simulink model "Cinematica_JA_reducido"  (Simulink 7.7)
settings: Solver=ode45  StartTime=0.0  StopTime=inf  RelTol=1e-3
libraries: vrlib x1
settings Model: Creator=JohnConstantine  LastModifiedBy=JohnConstantine

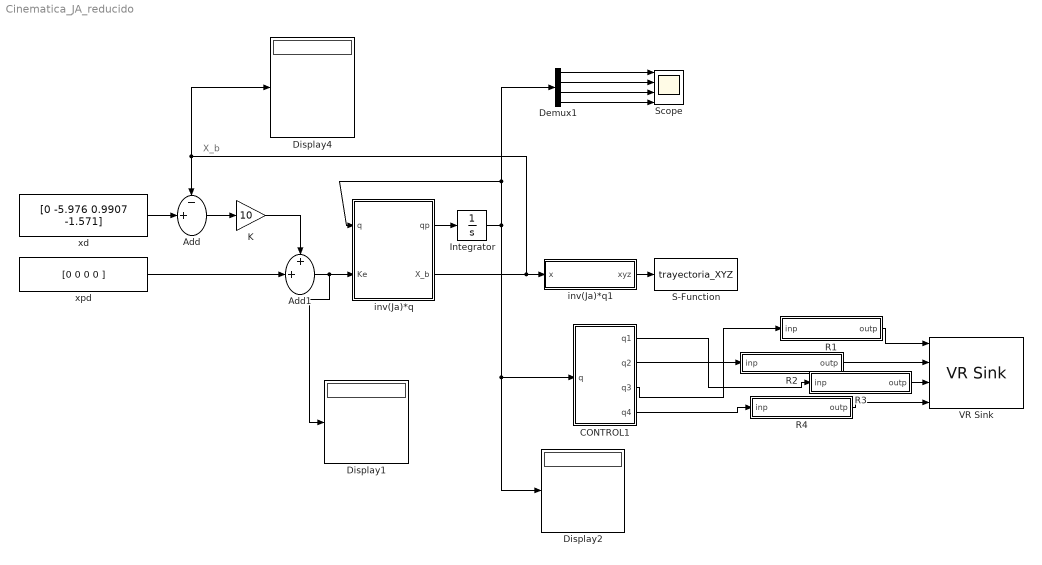
== system Cinematica_JA_reducido ==
  note: X_b
  Add : Sum  Inputs=-+|
  Add1 : Sum  Inputs=++|
  CONTROL1 : Stateflow chart  TreatAsAtomicUnit=on
  Demux1 : Demux
  Display1 : Display
  Display2 : Display
  Display4 : Display
  Integrator : Integrator  InitialCondition=[.001 .001 .001 .001]
  K : Gain  Gain=10
  R1 : Stateflow chart  TreatAsAtomicUnit=on
  R2 : Stateflow chart  TreatAsAtomicUnit=on
  R3 : Stateflow chart  TreatAsAtomicUnit=on
  R4 : Stateflow chart  TreatAsAtomicUnit=on
  S-Function : S-Function  FunctionName=trayectoria_XYZ  Parameters=[-7 7 -7 7 -7 7]  EnableBusSupport=off
  Scope : Scope  NumInputPorts=4
      settings: YMin=-0.2~0~0~-0.5  YMax=0.9~2.25~2~0.5
  VR Sink : vrlib/VR Sink  SampleTime=0.1  ViewEnable=on  RemoteChange=off  RemoteView=on  FieldsWritten=Q1.translation.3.1.1.double#Q2.rotation.4.1.1.double#Q3.rotation.4.1.1.double#Q4.rotation.4.1.1.double  WorldFileName=DedoCAD.WRL  AutoView=off  VideoDimensions=[]
  inv(Ja)*q : Stateflow chart  TreatAsAtomicUnit=on
  inv(Ja)*q1 : Stateflow chart  TreatAsAtomicUnit=on
  xd : Constant  Value=[0 -5.976 0.9907 -1.571]
  xpd : Constant  Value=[0 0 0 0 ]
  wires:
  Add/1 -> K/1
  xd/1 -> Add/2
  K/1 -> Add1/1
  xpd/1 -> Add1/2
  Add1/1 -> Display1/1, inv(Ja)*q/2(Ke)
  Integrator/1 -> inv(Ja)*q/1(q), Demux1/1, CONTROL1/1(q), Display2/1
  inv(Ja)*q/2(X_b) -> Add/1, Display4/1, inv(Ja)*q1/1(x)
  Demux1/1 -> Scope/1
  Demux1/2 -> Scope/2
  Demux1/3 -> Scope/3
  Demux1/4 -> Scope/4
  inv(Ja)*q1/1(xyz) -> S-Function/1
  R1/1(outp) -> VR Sink/1
  R2/1(outp) -> VR Sink/2
  R3/1(outp) -> VR Sink/3
  R4/1(outp) -> VR Sink/4
  CONTROL1/2(q2) -> R2/1(inp)
  CONTROL1/4(q4) -> R4/1(inp)
  CONTROL1/3(q3) -> R1/1(inp)
  CONTROL1/1(q1) -> R3/1(inp)
  inv(Ja)*q/1(qp) -> Integrator/1

== matlab function inv(Ja)*q1 ==
  data: x input double; xyz output double
function xyz   = Control(x)
X=x(1);
Y=x(2);
Z=x(3);
al=x(4);

xyz=[X Y Z]

== matlab function inv(Ja)*q ==
  data: q input double; qp output double; X_b output double; Ke input double
function [qp,X_b]  = Control(q,Ke)
q1=q(1);
q2=q(2);
q3=q(3);
q4=q(4);

% x1=Xpd_b_Ke(1);
% x2=Xpd_b_Ke(2);
% x3=Xpd_b_Ke(3);
% x4=Xpd_b_Ke(4);


qt=[q1 q2 q3 q4].'
%xpd_b_ke=[x1 x2 x3 x4].'

%% unidades en centimetros
d2=1.20349;
a2=.9907;
a3=.8862;
a4=1.5;
a5=.8862;
a6=1.5;

%%%%%%%%%%%%%%%%%%%%%%%%%%%%%%%%%
%%% Modelo geometrico directo %%%
%%%%%%%%%%%%%%%%%%%%%%%%%%%%%%%%%

 H=[ -cos(q3 + q4)*sin(q2),  sin(q3 + q4)*sin(q2), cos(q2),                                         -sin(q2)*(a2 + a5*cos(q3 + q4) + a6*cos(q3 + q4) + a3*cos(q3) + a4*cos(q3));...
               -sin(q3 + q4),         -cos(q3 + q4),       0,                                                  - d2 - a5*sin(q3 + q4) - a6*sin(q3 + q4) - a3*sin(q3) - a4*sin(q3);...
        cos(q3 + q4)*cos(q2), -sin(q3 + q4)*cos(q2), sin(q2), q1 + a2*cos(q2) + cos(q2)*cos(q3)*(a3 + a4) - cos(q2)*sin(q3)*sin(q4)*(a5 + a6) + cos(q2)*cos(q3)*cos(q4)*(a5 + a6);...
                           0,                     0,       0,                                                                                                                  1];
                                                                                                                                                                                                                                  
Pxyz=[H(1,4) H(2,4) H(3,4)].';

%%%%%%%%%%%%%%%%%%%%%%%%%%
%%% MATRIZ DE ROTACIÓN %%%
%%%%%%%%%%%%%%%%%%%%%%%%%%

R=[ -cos(q3 + q4)*sin(q2),  sin(q3 + q4)*sin(q2), cos(q2);
              -sin(q3 + q4),         -cos(q3 + q4),       0;
      cos(q3 + q4)*cos(q2), -sin(q3 + q4)*cos(q2), sin(q2)];

%%%%%%%%%%%%%%%%%%%%%%%%%%%%%%%%%%%%%%%%%%%%%%%%%%%%%%%%%%%%%%%%%%%%%%%%%%%%%%%%%%%%%%%%%%%%%%%%%%%%%%%%%%%%%%%%%%%%%%%%%%%%%%%%%%%%%%%%
%% variables para calcular alpha, gamma y theta.                                                                                     %%%
%% De los angulos RPY.  Las posiciones de la matriz de rotacion de los angulos de EULER y RPY para el calculo de alpha, gamma, theta %%%
%%%%%%%%%%%%%%%%%%%%%%%%%%%%%%%%%%%%%%%%%%%%%%%%%%%%%%%%%%%%%%%%%%%%%%%%%%%%%%%%%%%%%%%%%%%%%%%%%%%%%%%%%%%%%%%%%%%%%%%%%%%%%%%%%%%%%%%%
%%%%%%%%%%%%%%%%%%%%%%%%%%%%%%%%%
%%% Angulos Roll, Pitch y Yaw %%%
%%%%%%%%%%%%%%%%%%%%%%%%%%%%%%%%%

 r21=R(2,1);
 r11=R(1,1);
 r31=R(3,1);
 r32=R(3,2);
 r33=R(3,3);
 
 th=atan2(r21,r11);%Z
 ga=atan2(-r31,sqrt(r32^2+r33^2)); %Y
 al=atan2(r32,r33);%X

  Theta=[al ga th].'; % valores de theta
 
%%%%%%%%%%%%%%%%%%%%%%%%%%%%%%%%%
%%% JACOBIANO DEL MANIPULADOR %%%
%%%%%%%%%%%%%%%%%%%%%%%%%%%%%%%%%

Jg =[ 0, -cos(q2)*(a2 + a5*cos(q3 + q4) + a6*cos(q3 + q4) + a3*cos(q3) + a4*cos(q3)),  sin(q2)*(a5*sin(q3 + q4) + a6*sin(q3 + q4) + a3*sin(q3) + a4*sin(q3)),  sin(q3 + q4)*sin(q2)*(a5 + a6);
      0,                                                                           0,          - a5*cos(q3 + q4) - a6*cos(q3 + q4) - a3*cos(q3) - a4*cos(q3),         -cos(q3 + q4)*(a5 + a6);
      1, -sin(q2)*(a2 + a5*cos(q3 + q4) + a6*cos(q3 + q4) + a3*cos(q3) + a4*cos(q3)), -cos(q2)*(a5*sin(q3 + q4) + a6*sin(q3 + q4) + a3*sin(q3) + a4*sin(q3)), -sin(q3 + q4)*cos(q2)*(a5 + a6);
      0,                                                                           0,                                                                cos(q2),                         cos(q2);
      0,                                                                          -1,                                                                      0,                               0;
      0,                                                                           0,                                                                sin(q2),                         sin(q2)];


%%%%%%%%%%%%%%%%%%%%%%%%%%%%%%%%%%%%%%%%%%%%%%%%%%%%%%
%%% MATRIZ DE TRANSFORMACION DE LOS ANGULOS DE RPY %%%
%%%%%%%%%%%%%%%%%%%%%%%%%%%%%%%%%%%%%%%%%%%%%%%%%%%%%%

Tphi =[ cos(ga)*cos(th), -sin(th), 0;
        cos(ga)*sin(th),  cos(th), 0;
               -sin(ga),        0, 1];
              
iTphi=inv(Tphi);

Ta_phi=[ eye(3)    zeros(3,3); %[I     0    ]
         zeros(3,3)   iTphi]   %[0 inv(Tphi)]
    
%%%%%%%%%%%%%%%%%%%%%%%%%%%%%
%%% Jacobiano analítico  %%%%
%%%%%%%%%%%%%%%%%%%%%%%%%%%%%

Ja=(Ta_phi*Jg) %ES UNA MATRIZ DE TAMAÑO 6x4

%Ja_b=[Ja(1:3,1) Ja(1:3,2) Ja(1:3,3) Ja(1:3,4);
     % Ja(6,1)   Ja(6,2)   Ja(6,3)   Ja(6,4)];
 
 %%%%%%%%%%%%%%%%%%%%%%%%%%%%%%%%%%%
 %%% Jacobiano analítico inverso %%%
 %%%%%%%%%%%%%%%%%%%%%%%%%%%%%%%%%%%
 

[U,S,V] = svd(Ja);
 %S_a=S(4,4);
 lambda = 0.01;
if (S(4,4) < lambda)
    J_ainv=(Ja.'*Ja+lambda*eye(4))\Ja.';
else 
    J_ainv = pinv(Ja);
end

%%%%%%%%%%%%%%%%%%%%%%%%%%
%%% Vector de posición %%%
%%%%%%%%%%%%%%%%%%%%%%%%%%

 X_b=[Pxyz;
     Theta];
% L=Xpd_b_Ke;
 qp=J_ainv\Ke;

== matlab function CONTROL1 ==
  data: q input double; q1 output double; q2 output double; q3 output double; q4 output double
function [q1,q2,q3,q4]= articulaciones(q)


q1=q(1);
q2=q(2);
q3=q(3);
q4=q(4);

== matlab function R1 ==
  data: inp input double; outp output double
function outp =rot1(inp)
outp=[inp 0 0];

== matlab function R2 ==
  data: inp input double; outp output double
function outp =rot1(inp)
outp=[0 1 0 inp];

== matlab function R3 ==
  data: inp input double; outp output double
function outp =rot1(inp)
outp=[0 0 1 inp];

== matlab function R4 ==
  data: inp input double; outp output double
function outp =rot1(inp)
outp=[0 0 1 inp];
